simulink model "Neuron"  (R2019a)
settings: Solver=VariableStepAuto  StartTime=0.0  StopTime=SimulationTime  FixedStep=theta  RelTol=1e-3
values from neighbouring files (symbols this model uses):
  C = 10e-6    (= 1e-05)    [SCR_par.m]    (also in main_singleRNR.m)
  Is = 25e-9    (= 2.5e-08)    [SCR_par.m]    (also in main_singleRNR.m)
  R1 = 100e3    (= 100000)    [SCR_par.m]    (also in main_singleRNR.m)
  R2 = 1000e3    (= 1000000)    [SCR_par.m]    (also in main_singleRNR.m)
  theta = para.theta    [SCR_par.m]    (also in main_singleRNR.m = 0.125)
settings Model: SimulationMode=accelerator  Creator=2251338L  LastModifiedBy=lxp55
settings SolverCC: ZeroCrossControl=DisableAll  ZeroCrossAlgorithm=Adaptive
settings DataIOCC: SaveOutput=off  SignalLogging=off  DSMLogging=off  SaveTime=off  ReturnWorkspaceOutputs=off
settings OptimizationCC: EfficientMapNaN2IntZero=off
settings DebuggingCC: ArithmeticOperatorsInVariantConditions=warning
settings HardwareCC: TargetBitPerPointer=64  TargetBitPerSizeT=64  TargetBitPerPtrDiffT=64  TargetLongLongMode=on  TargetIntDivRoundTo=Zero  TargetEndianess=LittleEndian  TargetWordSize=64  TargetHWDeviceType=MATLAB Host  ProdEqTarget=off
settings CodeAppCC: MaxIdLength=128
settings GRTTargetCC: TargetLangStandard=C89/C90 (ANSI)  GRTInterface=on

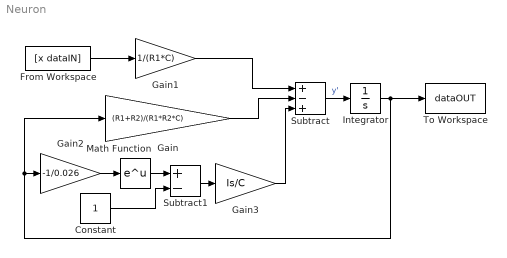
== system Neuron ==
  Constant : Constant
  From Workspace : FromWorkspace  VariableName=[x dataIN]  SampleTime=theta
  Gain : Gain  Gain=(R1+R2)/(R1*R2*C)
  Gain1 : Gain  Gain=1/(R1*C)
  Gain2 : Gain  Gain=-1/0.026
  Gain3 : Gain  Gain=Is/C
  Integrator : Integrator
  Math Function : Math  SaturateOnIntegerOverflow=on
  Subtract : Sum  Inputs=+-+
  Subtract1 : Sum  Inputs=+-
  To Workspace : ToWorkspace  VariableName=dataOUT  SampleTime=theta
  wires:
  Gain/1 -> Subtract/2
  Gain1/1 -> Subtract/1
  Subtract/1 -> Integrator/1  "y'"
  From Workspace/1 -> Gain1/1
  Gain2/1 -> Math Function/1
  Math Function/1 -> Subtract1/1
  Constant/1 -> Subtract1/2
  Subtract1/1 -> Gain3/1
  Integrator/1 -> To Workspace/1, Gain2/1, Gain/1
  Gain3/1 -> Subtract/3
